simulink model "ASSIGN_pe_q5"  (R2025b)
settings: Solver=VariableStepAuto  StartTime=0.0  StopTime=0.1  RelTol=1e-3
libraries: spsThyristorLib x8, spsRMSLib x4, spsVoltageMeasurementLib x4, spsACVoltageSourceLib x2, spsCurrentMeasurementLib x2, spsMeanLib x2, spsSeriesRLCBranchLib x2, spsDiodeLib x1, sps_lib x1
settings Model: Creator=Luqmaan  LastModifiedBy=Luqmaan

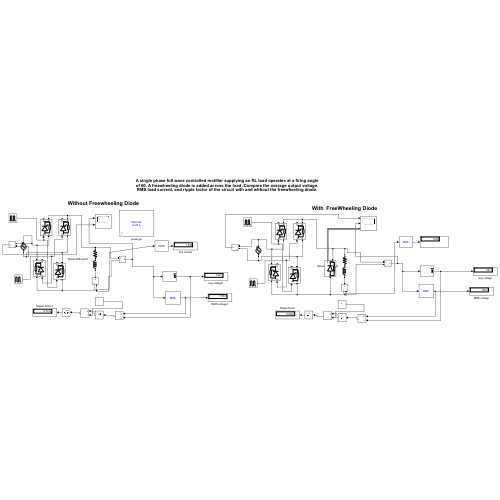
[thumbnail: Simulink's stored preview of the top-level diagram]
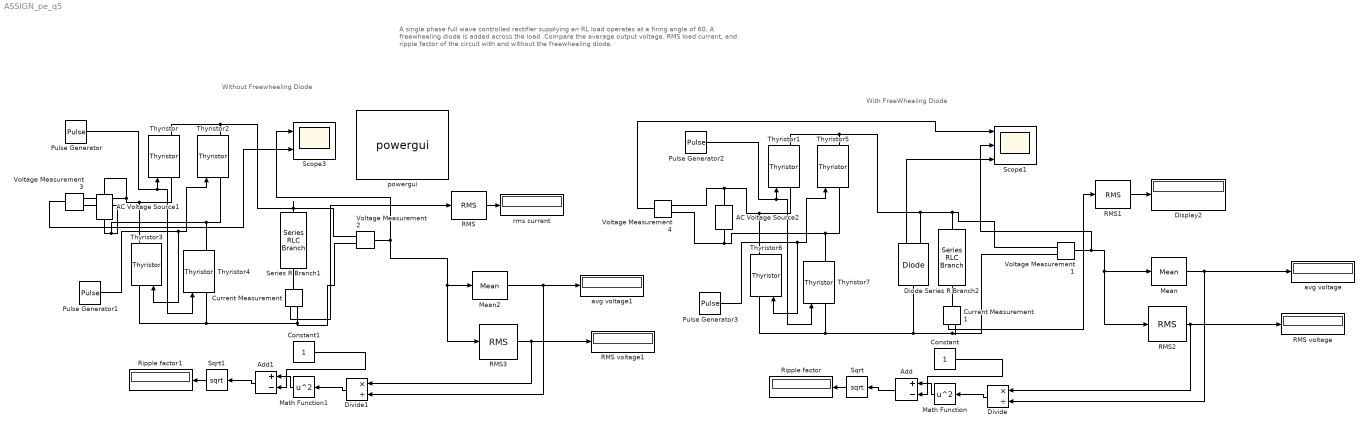
== system ASSIGN_pe_q5 ==
  note: With FreeWheeling Diode
  note: Without Freewheeling Diode
  note: A single phase full wave controlled rectifier supplying an RL load operates at a firing angle of 60. A freewheeling diode is added across the load .Compare the average output voltage. RMS load current, and ripple factor of the circuit with and wlthout the freewheeling diode.
  AC Voltage Source1 : spsACVoltageSourceLib/AC Voltage Source  Amplitude=230  Phase=0  Frequency=50  SampleTime=0  Measurements=None  BusType=swing  Pref=10e3  Qref=0  Qmin=-inf  Qmax=+inf
  AC Voltage Source2 : spsACVoltageSourceLib/AC Voltage Source  Amplitude=230  Phase=0  Frequency=50  SampleTime=0  Measurements=None  BusType=swing  Pref=10e3  Qref=0  Qmin=-inf  Qmax=+inf
  Add : Sum  Inputs=+-
  Add1 : Sum  Inputs=+-
  Constant : Constant
  Constant1 : Constant
  Current Measurement : spsCurrentMeasurementLib/Current Measurement  PhasorSimulation=off  OutputType=Complex  PSBequivalent=0
  Current Measurement1 : spsCurrentMeasurementLib/Current Measurement  PhasorSimulation=off  OutputType=Complex  PSBequivalent=0
  Diode : spsDiodeLib/Diode  Ron=0.001  Lon=0  Vf=0.8  IC=0  UseSnubber=0  Rs=500  Cs=250e-9  Measurements=on
  Display2 : Display
  Divide : Product  Inputs=*/
  Divide1 : Product  Inputs=*/
  Math Function : Math  Operator=square
  Math Function1 : Math  Operator=square
  Mean : spsMeanLib/Mean  Freq=60  Vinit=0  Ts=0
  Mean2 : spsMeanLib/Mean  Freq=60  Vinit=0  Ts=0
  Pulse Generator : DiscretePulseGenerator  PulseType=Time based  Period=0.02  PulseWidth=10  PhaseDelay=60*(0.02/360)
  Pulse Generator1 : DiscretePulseGenerator  PulseType=Time based  Period=0.02  PulseWidth=10  PhaseDelay=60*(0.02/360) + 0.01
  Pulse Generator2 : DiscretePulseGenerator  PulseType=Time based  Period=0.02  PulseWidth=10  PhaseDelay=60*(0.02/360)
  Pulse Generator3 : DiscretePulseGenerator  PulseType=Time based  Period=0.02  PulseWidth=10  PhaseDelay=60*(0.02/360) + 0.01
  RMS{,1..3} (4 alike) : spsRMSLib/RMS  TrueRMS=on  Freq=60  RMSInit=120  Ts=0
  RMS voltage : Display
  RMS voltage1 : Display
  Ripple factor : Display
  Ripple factor1 : Display
  Scope1 : Scope  NumInputPorts=3
      settings: ActiveDisplayYMinimum=-287.5  ActiveDisplayYMaximum=287.5
  Scope3 : Scope  NumInputPorts=2
      settings: ActiveDisplayYMinimum=-78.035854065604326  ActiveDisplayYMaximum=262.44539250348765
  Series R Branch1 : spsSeriesRLCBranchLib/Series RLC Branch  LConnTagsString=__new0  RConnTagsString=__new0  BranchType=RL  Resistance=100  Inductance=0.05  SetiL0=off  InitialCurrent=0  Capacitance=inf  Setx0=off  InitialVoltage=0  Measurements=None
  Series R Branch2 : spsSeriesRLCBranchLib/Series RLC Branch  LConnTagsString=__new0  RConnTagsString=__new0  BranchType=RL  Resistance=100  Inductance=0.05  SetiL0=off  InitialCurrent=0  Capacitance=inf  Setx0=off  InitialVoltage=0  Measurements=None
  Sqrt : Sqrt
  Sqrt1 : Sqrt
  Thyristor{,1..7} (8 alike) : spsThyristorLib/Thyristor  Ron=0.001  Lon=0  Vf=0.8  IC=0  Rs=500  Cs=250e-9  Measurements=on
  Voltage Measurement{1..4} (4 alike) : spsVoltageMeasurementLib/Voltage Measurement  PhasorSimulation=off  OutputType=Complex  PSBequivalent=0
  avg voltage : Display
  avg voltage1 : Display
  powergui : sps_lib/powergui  Priority=1  SimulationMode=Discrete  SampleTime=1e-5  frequency=60  Iterations=50  frequencyindice=50  Pbase=100e6  ErrMax=1e-4  UnitsV=kV  UnitsW=MW  buscounter=0  FunctionMessages=off  echomessages=off  EnableUseOfTLC=off  CurrentSourceSwitches=off  DisableSnubberDevices=off  DisableRonSwitches=off  DisableVfSwitches=off  DisplayEquations=off  AutomaticDiscreteSolvers=off  SolverType=Tustin/Backward Euler (TBE)  Interpol=off  ExternalGateDelay=off  methode=off  Ts=100  x0status=blocks  SPID=on  SwTol=0  HookPort=off  NonlinearTolerance=1e-4  nMaxIteration=100  ContinueOnMaxIteration=off  RestoreLinks=warning  ResistiveCurrentMeasurement=off  Frange=[0:2:500]  Ylog=off  Xlog=on  ShowGrid=off  save=off  variable=ZData  structure=0  ZoomFFT=off  StartTime=0.0  cycles=1  DisplayStyle=1  fundamental=60  FreqAxis=off  MaxFrequency=1000  frequencyindicesteady=1  RmsSteady=1  display=off
  rms current : Display
  wires:
  Pulse Generator/1 -> Thyristor4/1, Thyristor/1
  Pulse Generator1/1 -> Thyristor2/1, Thyristor3/1
  Voltage Measurement3/1 -> Scope3/2
  Voltage Measurement2/1 -> RMS3/1, Mean2/1, Scope3/1
  Pulse Generator2/1 -> Thyristor7/1, Thyristor1/1
  Pulse Generator3/1 -> Thyristor5/1, Thyristor6/1
  Voltage Measurement4/1 -> Scope1/1
  Voltage Measurement1/1 -> RMS2/1, Mean/1, Scope1/2
  Diode/1 -> Scope1/3
  Current Measurement/1 -> RMS/1
  RMS/1 -> rms current/1
  Current Measurement1/1 -> RMS1/1
  RMS1/1 -> Display2/1
  RMS2/1 -> RMS voltage/1, Divide/1
  Divide/1 -> Math Function/1
  Math Function/1 -> Add/1
  Constant/1 -> Add/2
  Add/1 -> Sqrt/1
  Sqrt/1 -> Ripple factor/1
  Add1/1 -> Sqrt1/1
  Sqrt1/1 -> Ripple factor1/1
  RMS3/1 -> Divide1/1, RMS voltage1/1
  Mean2/1 -> avg voltage1/1, Divide1/2
  Divide1/1 -> Math Function1/1
  Constant1/1 -> Add1/2
  Math Function1/1 -> Add1/1
  Mean/1 -> avg voltage/1, Divide/2
  connections:
  Thyristor2/LConn1 -- Thyristor4/RConn1 -- AC Voltage Source1/LConn1 -- Voltage Measurement3/LConn1
  Thyristor3/RConn1 -- AC Voltage Source1/RConn1 -- Voltage Measurement3/LConn2 -- Thyristor/LConn1
  Thyristor2/RConn1 -- Thyristor/RConn1 -- Voltage Measurement2/LConn1 -- Series R Branch1/LConn1
  Thyristor3/LConn1 -- Current Measurement/RConn1 -- Voltage Measurement2/LConn2 -- Thyristor4/LConn1
  AC Voltage Source2/LConn1 -- Voltage Measurement4/LConn1 -- Thyristor7/RConn1 -- Thyristor5/LConn1
  Thyristor6/RConn1 -- AC Voltage Source2/RConn1 -- Voltage Measurement4/LConn2 -- Thyristor1/LConn1
  Thyristor5/RConn1 -- Diode/RConn1 -- Voltage Measurement1/LConn1 -- Series R Branch2/LConn1 -- Thyristor1/RConn1
  Thyristor6/LConn1 -- Diode/LConn1 -- Current Measurement1/RConn1 -- Voltage Measurement1/LConn2 -- Thyristor7/LConn1
  Series R Branch1/RConn1 -- Current Measurement/LConn1
  Series R Branch2/RConn1 -- Current Measurement1/LConn1
